simulink model "SysModel_ADRC"  (R2018a)
settings: Solver=ode4  StartTime=0.0  StopTime=10.0  RelTol=1e-3
settings Model: Creator=Risky Jr  LastModifiedBy=Risky Jr

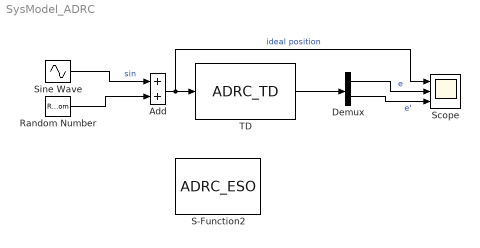
== system SysModel_ADRC ==
  Add : Sum
  Demux : Demux  Outputs=2
  Random Number : RandomNumber  Variance=0.1  SampleTime=0.001
  S-Function2 : S-Function  FunctionName=ADRC_ESO  SFunctionDeploymentMode=off  EnableBusSupport=off
  Scope : Scope  NumInputPorts=3
  Sine Wave : Sin  Frequency=62.8  SampleTime=1e-3
  TD : S-Function  FunctionName=ADRC_TD  Parameters=5e-3,1e4  SFunctionDeploymentMode=off  EnableBusSupport=off
  wires:
  Sine Wave/1 -> Add/1  "sin"
  Random Number/1 -> Add/2
  Add/1 -> Scope/1, TD/1  "ideal position"
  TD/1 -> Demux/1
  Demux/2 -> Scope/3  "e'"
  Demux/1 -> Scope/2  "e"
